simulink subsystem "startOLAECore"  (R2021a)
settings: Solver=VariableStepAuto  StartTime=0.0  StopTime=10.0  RelTol=1e-3
settings Model: Creator=noraw  LastModifiedBy=noraw

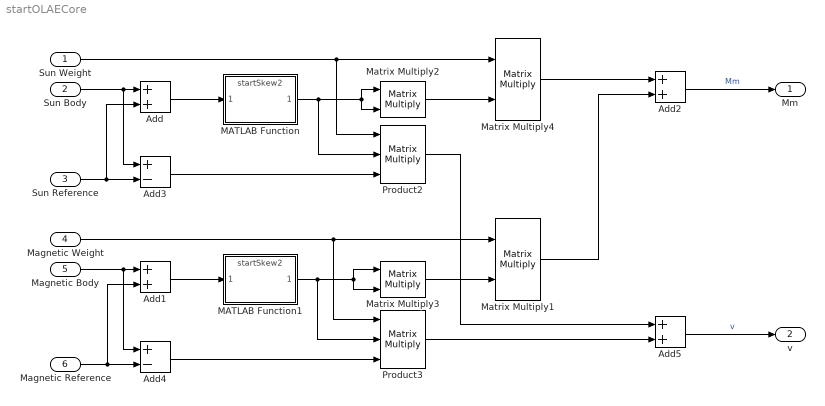
== system startOLAECore ==
  Sun Weight : Inport  PortDimensions=[3 3]
  Sun Body : Inport  Port=2  PortDimensions=3
  Sun Reference : Inport  Port=3  PortDimensions=3
  Magnetic Weight : Inport  Port=4  PortDimensions=[3 3]
  Magnetic Body : Inport  Port=5  PortDimensions=3
  Magnetic Reference : Inport  Port=6  PortDimensions=3
  Add{,1..2,5} (4 alike) : Sum
  Add3 : Sum  Inputs=+-
  Add4 : Sum  Inputs=+-
  MATLAB Function : ModelReference  ModelNameDialog=startSkew2  SimulationMode=Normal  ModelReferenceVersion=3.29
  MATLAB Function1 : ModelReference  ModelNameDialog=startSkew2  SimulationMode=Normal  ModelReferenceVersion=3.29
  Matrix Multiply{1..4} (4 alike) : Product  Multiplication=Matrix(*)
  Product2 : Product  Inputs=3  Multiplication=Matrix(*)
  Product3 : Product  Inputs=3  Multiplication=Matrix(*)
  Mm : Outport
  v : Outport  Port=2
  wires:
  Add3/1 -> Product2/3
  Sun Reference/1 -> Add/2, Add3/2
  Add5/1 -> v/1  "v"
  Add2/1 -> Mm/1  "Mm"
  Add4/1 -> Product3/3
  Sun Body/1 -> Add/1, Add3/1
  Matrix Multiply3/1 -> Matrix Multiply1/2
  Magnetic Body/1 -> Add1/1, Add4/1
  Matrix Multiply4/1 -> Add2/1
  Matrix Multiply1/1 -> Add2/2
  Add1/1 -> MATLAB Function1/1
  Product2/1 -> Add5/1
  Magnetic Reference/1 -> Add4/2, Add1/2
  Product3/1 -> Add5/2
  MATLAB Function1/1 -> Product3/2, Matrix Multiply3/2, Matrix Multiply3/1
  Matrix Multiply2/1 -> Matrix Multiply4/2
  Magnetic Weight/1 -> Product3/1, Matrix Multiply1/1
  Add/1 -> MATLAB Function/1
  Sun Weight/1 -> Product2/1, Matrix Multiply4/1
  MATLAB Function/1 -> Product2/2, Matrix Multiply2/1, Matrix Multiply2/2
